simulink model "Simulink_FINAL_EXAM_A01636406"  (R2020a)
settings: Solver=VariableStepAuto  StartTime=0.0  StopTime=30  RelTol=1e-3
undefined symbols (not defined in the file): A1, A2, A3, B1, B2, B3, C1, C2, C3, k1_coup, K2, k3_coup, K_1, K_3, kc, kd, ki, L_1
libraries: cstblocks x2
settings Model: Creator=beto1  LastModifiedBy=beto1

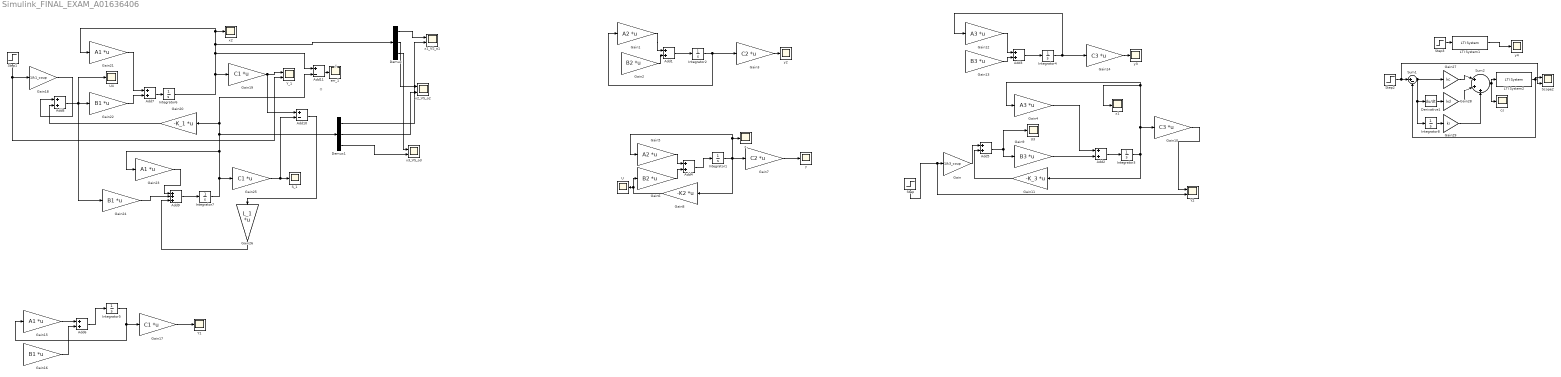
== system Simulink_FINAL_EXAM_A01636406 ==
  note: X
  note: O
  Add{1..8} (8 alike) : Sum
  Add10 : Sum  Inputs=+-
  Add11 : Sum  Inputs=+-
  Add9 : Sum  Inputs=+++
  Demux : Demux  Outputs=3
  Demux1 : Demux  Outputs=3
  Derivative1 : Derivative
  Gain : Gain  Gain=1/k3_coup
  Gain1 : Gain  Gain=A2  Multiplication=Matrix(K*u)
  Gain10 : Gain  Gain=C3  Multiplication=Matrix(K*u)
  Gain11 : Gain  Gain=-K_3  Multiplication=Matrix(K*u)
  Gain12 : Gain  Gain=A3  Multiplication=Matrix(K*u)
  Gain13 : Gain  Gain=B3  Multiplication=Matrix(K*u)
  Gain14 : Gain  Gain=C3  Multiplication=Matrix(K*u)
  Gain15 : Gain  Gain=A1  Multiplication=Matrix(K*u)
  Gain16 : Gain  Gain=B1  Multiplication=Matrix(K*u)
  Gain17 : Gain  Gain=C1  Multiplication=Matrix(K*u)
  Gain18 : Gain  Gain=1/k1_coup
  Gain19 : Gain  Gain=C1  Multiplication=Matrix(K*u)
  Gain2 : Gain  Gain=B2  Multiplication=Matrix(K*u)
  Gain20 : Gain  Gain=-K_1  Multiplication=Matrix(K*u)
  Gain21 : Gain  Gain=A1  Multiplication=Matrix(K*u)
  Gain22 : Gain  Gain=B1  Multiplication=Matrix(K*u)
  Gain23 : Gain  Gain=A1  Multiplication=Matrix(K*u)
  Gain24 : Gain  Gain=B1  Multiplication=Matrix(K*u)
  Gain25 : Gain  Gain=C1  Multiplication=Matrix(K*u)
  Gain26 : Gain  Gain=L_1  Multiplication=Matrix(K*u)
  Gain27 : Gain  Gain=kc
  Gain28 : Gain  Gain=kd
  Gain29 : Gain  Gain=ki
  Gain3 : Gain  Gain=C2  Multiplication=Matrix(K*u)
  Gain4 : Gain  Gain=A3  Multiplication=Matrix(K*u)
  Gain5 : Gain  Gain=A2  Multiplication=Matrix(K*u)
  Gain6 : Gain  Gain=B2  Multiplication=Matrix(K*u)
  Gain7 : Gain  Gain=C2  Multiplication=Matrix(K*u)
  Gain8 : Gain  Gain=-K2  Multiplication=Matrix(K*u)
  Gain9 : Gain  Gain=B3  Multiplication=Matrix(K*u)
  Integrator{1..6} (6 alike) : Integrator  InitialCondition=[1 2 3]
  Integrator7 : Integrator
  Integrator8 : Integrator
  LTI System1 : cstblocks/LTI System  sys=G4  IC=[]
  LTI System2 : cstblocks/LTI System  sys=G4  IC=[]
  S_1 : Scope
  Scope2 : Scope  NumInputPorts=2
  Step : Step  Time=0  After=22  SampleTime=0
  Step1 : Step  Time=0  After=11  SampleTime=0
  Step2 : Step  Time=0  After=33  SampleTime=0
  Step3 : Step  Time=0  After=33  SampleTime=0
  Sum1 : Sum  Inputs=|+-
  Sum2 : Sum  Inputs=|+++
  U : Scope
  U3 : Scope
  U4 : Scope
  Y1 : Scope
  Y2 : Scope  NumInputPorts=2
  Y_1 : Scope  NumInputPorts=2
  cs : Scope
  err_1 : Scope
  x : Scope
  x1 : Scope
  x1_VS_o1 : Scope  NumInputPorts=2
  x2 : Scope
  x2_VS_o2 : Scope  NumInputPorts=2
  x3_VS_o3 : Scope  NumInputPorts=2
  y{,2..4} (4 alike) : Scope
  wires:
  Add8/1 -> U4/1, Gain22/1, Gain24/1
  Integrator6/1 -> Add11/1, Demux/1, Gain21/1, x2/1, Gain19/1
  Gain24/1 -> Add9/2
  Gain25/1 -> S_1/1, Add10/2
  Gain20/1 -> Add8/2
  Add10/1 -> Gain26/1
  Demux1/2 -> x2_VS_o2/2
  Add11/1 -> err_1/1
  Step1/1 -> Y_1/2, Gain18/1
  Demux/1 -> x1_VS_o1/1
  Demux/3 -> x3_VS_o3/1
  Add7/1 -> Integrator6/1
  Gain21/1 -> Add7/1
  Integrator7/1 -> Gain25/1, Add11/2, Gain20/1, Demux1/1, Gain23/1
  Gain23/1 -> Add9/1
  Gain18/1 -> Add8/1
  Gain26/1 -> Add9/3
  Demux1/3 -> x3_VS_o3/2
  Add9/1 -> Integrator7/1
  Gain19/1 -> Add10/1, Y_1/1
  Gain22/1 -> Add7/2
  Demux/2 -> x2_VS_o2/1
  Demux1/1 -> x1_VS_o1/2
  Gain16/1 -> Add6/2
  Gain17/1 -> Y1/1
  Integrator5/1 -> Gain15/1, Gain17/1
  Gain15/1 -> Add6/1
  Add6/1 -> Integrator5/1
  Integrator1/1 -> Gain7/1, Gain5/1, x/1, Gain8/1
  Gain7/1 -> y/1
  Gain1/1 -> Add1/1
  Add1/1 -> Integrator2/1
  Gain3/1 -> y2/1
  Gain8/1 -> U/1, Gain6/1
  Gain2/1 -> Add1/2
  Integrator2/1 -> Gain1/1, Gain3/1
  Add4/1 -> Integrator1/1
  Gain5/1 -> Add4/1
  Gain6/1 -> Add4/2
  Add3/1 -> Integrator4/1
  Gain14/1 -> y3/1
  Gain13/1 -> Add3/2
  Gain10/1 -> Y2/1
  Integrator3/1 -> x1/1, Gain4/1, Gain10/1, Gain11/1
  Gain11/1 -> Add5/2
  Gain12/1 -> Add3/1
  Integrator4/1 -> Gain14/1, Gain12/1
  Add2/1 -> Integrator3/1
  Gain9/1 -> Add2/2
  Add5/1 -> U3/1, Gain9/1
  Step/1 -> Y2/2, Gain/1
  Gain/1 -> Add5/1
  Gain4/1 -> Add2/1
  Step3/1 -> LTI System1/1
  LTI System1/1 -> y4/1
  Gain27/1 -> Sum2/1
  Step2/1 -> Scope2/2, Sum1/1
  Gain28/1 -> Sum2/2
  Sum1/1 -> Integrator8/1, Derivative1/1, Gain27/1
  Sum2/1 -> cs/1, LTI System2/1
  Derivative1/1 -> Gain28/1
  Gain29/1 -> Sum2/3
  Integrator8/1 -> Gain29/1
  LTI System2/1 -> Sum1/2, Scope2/1
